simulink model "motorsim1"  (R2018b)
settings: Solver=ode45  StartTime=0.0  StopTime=0.5  FixedStep=1e-4  MaxStep=1e-4  RelTol=1e-3  EnableMultiTasking=on
settings Model: Creator=tcraddoc  LastModifiedBy=rbarve
settings DataIOCC: LimitDataPoints=on  SaveFormat=Array  SignalLoggingSaveFormat=ModelDataLogs  SignalLoggingName=sigsOut
settings OptimizationCC: BooleanDataType=off  LifeSpan=inf
settings DebuggingCC: SaveWithParameterizedLinksMsg=none  UnderspecifiedInitializationDetection=Classic  MergeDetectMultiDrivingBlocksExec=none  SignalResolutionControl=TryResolveAllWithWarning  MultiTaskDSMMsg=warning  MultiTaskCondExecSysMsg=none  SFUnexpectedBacktrackingDiag=warning  SFNoUnconditionalDefaultTransitionDiag=warning  SFExecutionAtInitializationDiag=none
settings HardwareCC: ProdBitPerPointer=32  ProdBitPerSizeT=32  ProdBitPerPtrDiffT=32  ProdLargestAtomicFloat=None  ProdIntDivRoundTo=Undefined  ProdEndianess=Unspecified  ProdWordSize=32  ProdHWDeviceType=32-bit Generic  TargetUnknown=on
settings ModelReferenceCC: PropagateSignalLabelsOutOfModel=off
settings SFSimCC: SimUseLocalCustomCode=off
settings RTWCC: RTWUseLocalCustomCode=off
settings CodeAppCC: StateflowObjectComments=on
settings GRTTargetCC: TargetLangStandard=C89/C90 (ANSI)  GeneratePreprocessorConditionals=Disable all  CombineOutputUpdateFcns=off  GRTInterface=on
settings ConfigComp: CovMetricSettings=dw  CovHtmlReporting=on  CovSaveCumulativeToWorkspaceVar=on  CovSaveSingleToWorkspaceVar=on  CovExternalEMLEnable=off

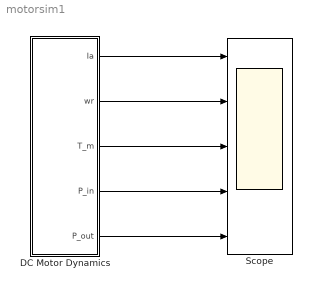
== system motorsim1 ==
  DC Motor Dynamics : Subsystem  mask{V=4, ra=2, Bm=0.00007009, Kv=0.037, J=9.6718e-05, Tstick=.00107}
      mask prompts: V "Va (Armature Voltage)"; ra "ra (Armature resistance)"; Bm "Bm (Coefficient of Friction)"; Kv "kv (voltage constant)"; J "J (Rotor moment of inertia)"; Tstick "Tstick ("Sticking" Torque)"
  Scope : Scope  NumInputPorts=5
      settings: AttributesFormatString=Click to see the plots
  wires:
  DC Motor Dynamics/1(Ia) -> Scope/1
  DC Motor Dynamics/2(wr) -> Scope/2
  DC Motor Dynamics/3(T_m) -> Scope/3
  DC Motor Dynamics/4(P_in) -> Scope/4
  DC Motor Dynamics/5(P_out) -> Scope/5

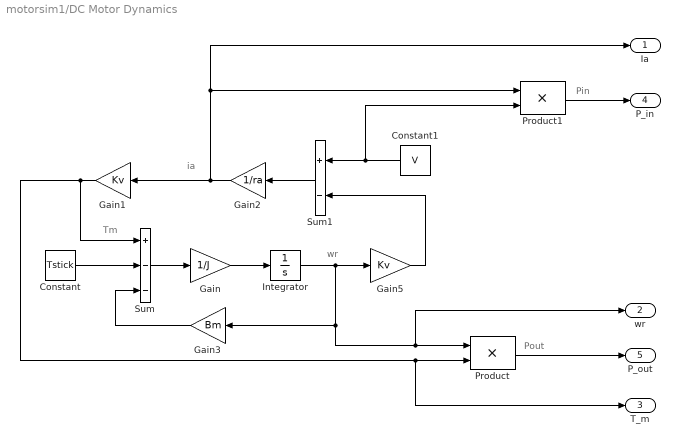
== system motorsim1/DC Motor Dynamics ==
  note: wr
  note: Tm
  note: ia
  note: Pout
  note: Pin
  Constant : Constant  Value=Tstick
  Constant1 : Constant  Value=V
  Gain : Gain  Gain=1/J  SaturateOnIntegerOverflow=on  OutDataTypeStr=Inherit: Same as input  ParamDataTypeStr=Inherit: Same as input
  Gain1 : Gain  Gain=Kv  SaturateOnIntegerOverflow=on  OutDataTypeStr=Inherit: Same as input  ParamDataTypeStr=Inherit: Same as input
  Gain2 : Gain  Gain=1/ra  SaturateOnIntegerOverflow=on  OutDataTypeStr=Inherit: Same as input  ParamDataTypeStr=Inherit: Same as input
  Gain3 : Gain  Gain=Bm  SaturateOnIntegerOverflow=on  OutDataTypeStr=Inherit: Same as input  ParamDataTypeStr=Inherit: Same as input
  Gain5 : Gain  Gain=Kv  SaturateOnIntegerOverflow=on  OutDataTypeStr=Inherit: Same as input  ParamDataTypeStr=Inherit: Same as input
  Integrator : Integrator
  Product : Product  SaturateOnIntegerOverflow=on  InputSameDT=on  OutDataTypeStr=Inherit: Same as first input
  Product1 : Product  SaturateOnIntegerOverflow=on  InputSameDT=on  OutDataTypeStr=Inherit: Same as first input
  Sum : Sum  Inputs=+--  SaturateOnIntegerOverflow=on  InputSameDT=on  OutDataTypeStr=Inherit: Same as first input
  Sum1 : Sum  Inputs=+-  SaturateOnIntegerOverflow=on  InputSameDT=on  OutDataTypeStr=Inherit: Same as first input
  Ia : Outport
  wr : Outport  Port=2
  T_m : Outport  Port=3
  P_in : Outport  Port=4
  P_out : Outport  Port=5
  wires:
  Sum/1 -> Gain/1
  Gain/1 -> Integrator/1
  Constant/1 -> Sum/2
  Gain1/1 -> Sum/1, Product/2, T_m/1
  Gain3/1 -> Sum/3
  Integrator/1 -> Gain5/1, Gain3/1, Product/1, wr/1
  Gain2/1 -> Gain1/1, Ia/1, Product1/1
  Sum1/1 -> Gain2/1
  Gain5/1 -> Sum1/2
  Product1/1 -> P_in/1
  Product/1 -> P_out/1
  Constant1/1 -> Product1/2, Sum1/1
